simulink model "b_half_bridge_average_value_with_diode"  (R2025b)
settings: Solver=VariableStepAuto  StartTime=0.0  StopTime=1/60  RelTol=1e-3
libraries: fl_lib x19, nesl_utility x8, ee_lib x2
settings Model: SimulationMode=accelerator  Creator=gdudgeon  LastModifiedBy=gdudgeon

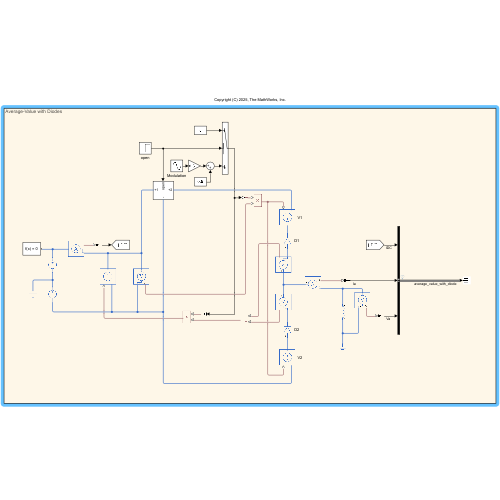
[thumbnail: Simulink's stored preview of the top-level diagram]
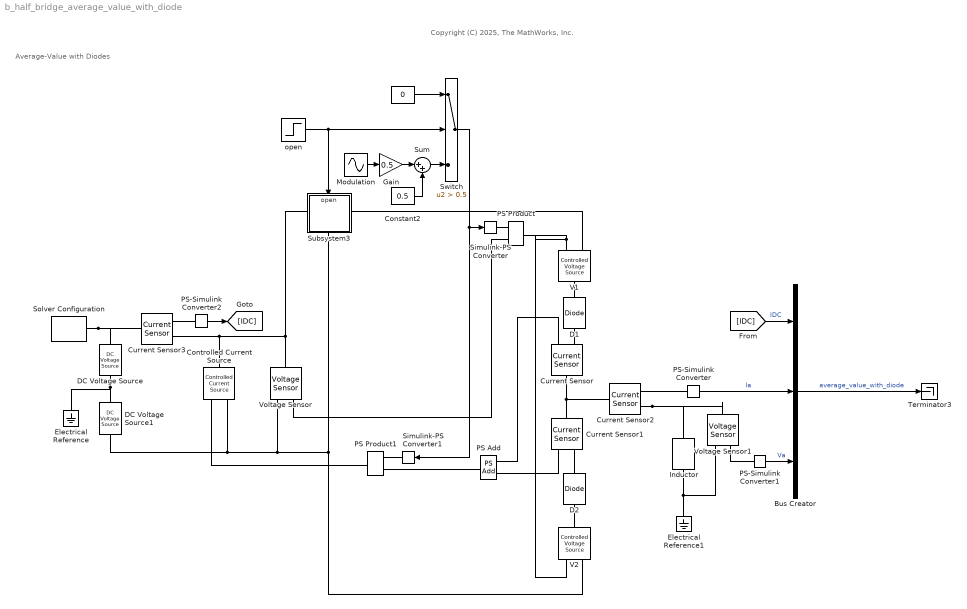
== system b_half_bridge_average_value_with_diode ==
  note: Copyright (C) 2025, The MathWorks, Inc.
  note: Average-Value with Diodes
  " " : Constant  Value=0  SampleTime=-1
  Bus Creator : BusCreator  Inputs=3
  Constant2 : Constant  Value=0.5  SampleTime=-1
  Controlled Current Source : fl_lib/Electrical/Electrical Sources/Controlled Current Source
  Current Sensor{,1..3} (4 alike) : fl_lib/Electrical/Electrical Sensors/Current Sensor
  D1 : fl_lib/Electrical/Electrical Elements/Diode  Vf=1e-3 V  Ron=1e-3 Ohm  Goff=1e-5 1/Ohm  i_specify=off  i_priority=None  i=0 A  i_nominal_specify=off  i_nominal_value=1  i_nominal_unit=A  v_specify=off  v_priority=None  v=0 V  v_nominal_specify=off  v_nominal_value=1  v_nominal_unit=V
  D2 : fl_lib/Electrical/Electrical Elements/Diode  Vf=1e-3 V  Ron=1e-3 Ohm  Goff=1e-5 1/Ohm  i_specify=off  i_priority=None  i=0 A  i_nominal_specify=off  i_nominal_value=1  i_nominal_unit=A  v_specify=off  v_priority=None  v=0 V  v_nominal_specify=off  v_nominal_value=1  v_nominal_unit=V
  DC Voltage Source : fl_lib/Electrical/Electrical Sources/DC Voltage Source  v0=50 V
  DC Voltage Source1 : fl_lib/Electrical/Electrical Sources/DC Voltage Source  v0=50 V
  Electrical Reference : fl_lib/Electrical/Electrical Elements/Electrical Reference
  Electrical Reference1 : fl_lib/Electrical/Electrical Elements/Electrical Reference
  Gain : Gain  Gain=0.5
  Inductor : fl_lib/Electrical/Electrical Elements/Inductor  l=0.01 H  r=1 Ohm  g=0 1/Ohm  i_specify=off  i_priority=None  i=0 A  i_nominal_specify=off  i_nominal_value=1  i_nominal_unit=A  v_specify=off  v_priority=High  v=0 V  v_nominal_specify=off  v_nominal_value=1  v_nominal_unit=V  i_L_specify=off  i_L_priority=High  i_L=0 A  i_L_nominal_specify=off  i_L_nominal_value=1  i_L_nominal_unit=A
  Modulation : Sin  Amplitude=0.8  Frequency=120*pi  SampleTime=0
  PS Add : fl_lib/Physical Signals/Functions/PS Add
  PS Product : fl_lib/Physical Signals/Functions/PS Product
  PS Product1 : fl_lib/Physical Signals/Functions/PS Product
  PS-Simulink Converter : nesl_utility/PS-Simulink Converter  PhysicalDomain=network_engine_domain  SubClassName=ps_output  LeftPortType=input  RightPortType=output  PseudoPeriodic=off  Frequencies=[]  VectorFormat=inherit  Unit=inherit  AffineConversion=off
  PS-Simulink Converter1 : nesl_utility/PS-Simulink Converter  PhysicalDomain=network_engine_domain  SubClassName=ps_output  LeftPortType=input  RightPortType=output  PseudoPeriodic=off  Frequencies=[]  VectorFormat=inherit  Unit=inherit  AffineConversion=off
  PS-Simulink Converter2 : nesl_utility/PS-Simulink Converter  PhysicalDomain=network_engine_domain  SubClassName=ps_output  LeftPortType=input  RightPortType=output  PseudoPeriodic=off  Frequencies=[]  VectorFormat=inherit  Unit=inherit  AffineConversion=off
  Simulink-PS Converter : nesl_utility/Simulink-PS Converter  PhysicalDomain=network_engine_domain  SubClassName=ps_input  LeftPortType=input  RightPortType=output  PseudoPeriodic=off  Frequencies=[]  NoiseDistribution=none  NoiseParameters=[]  Unit=1  AffineConversion=off  FilteringAndDerivatives=provide  SimscapeFilterOrder=1  InputFilterTimeConstant=0.001  UdotUserProvided=0
  Simulink-PS Converter1 : nesl_utility/Simulink-PS Converter  PhysicalDomain=network_engine_domain  SubClassName=ps_input  LeftPortType=input  RightPortType=output  PseudoPeriodic=off  Frequencies=[]  NoiseDistribution=none  NoiseParameters=[]  Unit=1  AffineConversion=off  FilteringAndDerivatives=provide  SimscapeFilterOrder=1  InputFilterTimeConstant=0.001  UdotUserProvided=0
  Solver Configuration : nesl_utility/Solver Configuration  PhysicalDomain=network_engine_domain  SubClassName=solver  LeftPortType=input  RightPortType=generic  Tones=[]  Harmonics=[]  SimulateNoise=off  Profile=off  UseLocalSampling=off  EnableSwitchedLinearOptims=on  FrequencyDomain=off  UseCCode=off  RelTol=0.001  AbsTol=0.001  MinStep=1e-09  ToWorkspace=off  RevertToSquareIcSolve=off  NumHomotopyIterations=100  PhasorMode=off  PhasorModeNumHarmonics=1  ConsistencySolver=NEWTON_XTOL_AFTER_FTOL  IndexReductionMethod=DerivativeReplacement  DoDC=off  ResidualTolerance=1e-09  ConsistencyTolSource=GLOBAL  ConsistencyAbsTol=0.001  ConsistencyRelTol=0.001  ConsistencyTolFactor=0.001  UseLocalSolver=on  LocalSolverChoice=NE_PARTITIONING_ADVANCER  ResolveIndetEquations=on  FunctionEvalNumThread=1  LocalSolverSampleTime=1e-6  DoFixedCost=off  MaxNonlinIter=3  MaxModeIter=2  ComputeImpulses=off  ImpulseIterations=2  LinearAlgebra=auto  LinearAlgebraNumThread=0  EquationFormulation=NE_TIME_EF  DelaysMemoryBudget=1024  AutomaticFiltering=off  FilteringTimeConstant=0.001  PartitionStorageMethod=AS_NEEDED  PartitionMemoryBudget=1024  PartitionMethod=ROBUST  MultibodyUseLocalSolver=off  MultibodyLocalSolverChoice=ODE1  MultibodyLocalSolverSampleTime=0.001
  Subsystem3 : Subsystem
      settings: PortSchema="{\"entries\":[{\"content\":{\"sides\":[{\"content\":{\"connectorIds\":[\"LConn1\"]},\"type\":\"ConnectorPlacement.EquallySpacedRectSide\",\"uuid\":\"88db1bd8-f64b-4165-8d2c-7cfa4014cba2\"},{\"content\":{\"connectorIds\":[\"RConn1\"],\"side\":\"RIGHT\"},\"type\":\"ConnectorPlacement.EquallySpacedRectSide\",\"uuid\":\"19f0c499-9eed-48d3-a8f5-fe9dad581b85\"},{\"content\":{\"connectorIds\":[\"In1\"],\"side\":\"TOP\"},\"type\":\"ConnectorPlacement.EquallySpacedRectSide\",\"uuid\":\"71d5fe89-ffc2-4430-819d-512bfd197a1c\"},{\"content\":{\"connectorIds\":[\"RConn2\"],\"side\":\"BOTTOM\"},\"type\":\"ConnectorPlacement.EquallySpacedRectSide\",\"uuid\":\"b828cb58-5f78-4b23-b8a0-147c7a9d81e7\"}]},\"type\":\"ConnectorPlacement.EquallySpacedConnector\",\"uuid\":\"64b174d4-80a0-4eb7-9a75-e3677787263f\"}],\"packageUris\":[\"http://schema.mathworks.com/mf0/Connector/R2020b\"],\"version\":\"1.0\"}"
  Sum : Sum  Inputs=|++
  Switch : Switch  Criteria=u2 > Threshold  Threshold=0.5  SaturateOnIntegerOverflow=off  InputSameDT=off
  Terminator3 : Terminator
  V1 : fl_lib/Electrical/Electrical Sources/Controlled Voltage Source
  V2 : fl_lib/Electrical/Electrical Sources/Controlled Voltage Source
  Voltage Sensor : fl_lib/Electrical/Electrical Sensors/Voltage Sensor
  Voltage Sensor1 : fl_lib/Electrical/Electrical Sensors/Voltage Sensor
  open : Step  After=0  SampleTime=0
  wires:
  Switch/1 -> Simulink-PS Converter1/1, Simulink-PS Converter/1
  " "/1 -> Switch/1
  [IDC] -> Bus Creator/1  "IDC"
  PS-Simulink Converter2/1 -> [IDC]
  open/1 -> Switch/2, Subsystem3/1(open)
  Bus Creator/1 -> Terminator3/1  "average_value_with_diode"
  PS-Simulink Converter1/1 -> Bus Creator/3  "Va"
  PS-Simulink Converter/1 -> Bus Creator/2  "Ia"
  Sum/1 -> Switch/3
  Modulation/1 -> Gain/1
  Constant2/1 -> Sum/2
  Gain/1 -> Sum/1
  connections:
  Solver Configuration/RConn1 -- DC Voltage Source/LConn1 -- Current Sensor3/LConn1
  Current Sensor3/RConn2 -- Controlled Current Source/LConn1 -- Subsystem3/LConn1 -- Voltage Sensor/LConn1
  Current Sensor2/LConn1 -- Current Sensor1/LConn1 -- Current Sensor/LConn1
  Electrical Reference1/LConn1 -- Inductor/RConn1 -- Voltage Sensor1/RConn2
  DC Voltage Source/RConn1 -- DC Voltage Source1/LConn1 -- Electrical Reference/LConn1
  Current Sensor2/RConn2 -- Inductor/LConn1 -- Voltage Sensor1/LConn1
  V1/RConn1 -- V2/RConn1 -- PS Product/RConn1
  Subsystem3/RConn2 -- V2/RConn2 -- Voltage Sensor/RConn2 -- DC Voltage Source1/RConn1 -- Controlled Current Source/RConn2
  Voltage Sensor/RConn1 -- PS Product/LConn2
  PS Add/LConn1 -- Current Sensor1/RConn1
  D2/LConn1 -- V2/LConn1
  Simulink-PS Converter/RConn1 -- PS Product/LConn1
  PS-Simulink Converter2/LConn1 -- Current Sensor3/RConn1
  D1/RConn1 -- V1/LConn1
  PS Product1/LConn1 -- PS Add/RConn1
  D1/LConn1 -- Current Sensor/RConn2
  PS Product1/RConn1 -- Controlled Current Source/RConn1
  PS-Simulink Converter1/LConn1 -- Voltage Sensor1/RConn1
  Subsystem3/RConn1 -- V1/RConn2
  Simulink-PS Converter1/RConn1 -- PS Product1/LConn2
  D2/RConn1 -- Current Sensor1/RConn2
  Current Sensor2/RConn1 -- PS-Simulink Converter/LConn1
  PS Add/LConn2 -- Current Sensor/RConn1

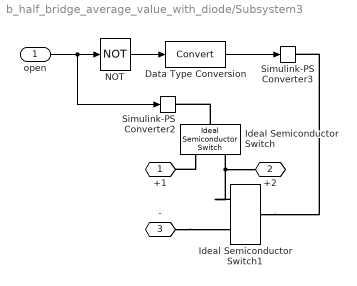
== system b_half_bridge_average_value_with_diode/Subsystem3 ==
  open : Inport
  Data Type Conversion : DataTypeConversion  SaturateOnIntegerOverflow=off  RndMeth=Floor
  Ideal Semiconductor Switch : ee_lib/Semiconductors & Converters/Ideal Semiconductor Switch  port_option=ee.enum.controlport.ps  Ron=1e-5 Ohm  Goff=1e-5 1/Ohm  Vth=0.5 V  diode_param=ee.enum.semiconductors.protectionDiode.external  diode_Vf=0.8 V  diode_Ron=0.001 Ohm  diode_Goff=1e-5 1/Ohm  diode_C=50e-9 F  diode_iRM=-235 A  diode_iF=300 A  diode_idot=-50 A/us  diode_trr_param=ee.enum.converters.diodetrr.trr_factor  diode_trr_factor=3  diode_trr=15 us  diode_Qrr=1500 s*uA
  Ideal Semiconductor Switch1 : ee_lib/Semiconductors & Converters/Ideal Semiconductor Switch  port_option=ee.enum.controlport.ps  Ron=1e-5 Ohm  Goff=1e-5 1/Ohm  Vth=0.5 V  diode_param=ee.enum.semiconductors.protectionDiode.external  diode_Vf=0.8 V  diode_Ron=0.001 Ohm  diode_Goff=1e-5 1/Ohm  diode_C=50e-9 F  diode_iRM=-235 A  diode_iF=300 A  diode_idot=-50 A/us  diode_trr_param=ee.enum.converters.diodetrr.trr_factor  diode_trr_factor=3  diode_trr=15 us  diode_Qrr=1500 s*uA
  NOT : Logic  Operator=NOT  IconShape=distinctive  AllPortsSameDT=off  OutDataTypeStr=boolean
  Simulink-PS Converter2 : nesl_utility/Simulink-PS Converter  PhysicalDomain=network_engine_domain  SubClassName=ps_input  LeftPortType=input  RightPortType=output  PseudoPeriodic=off  Frequencies=[]  NoiseDistribution=none  NoiseParameters=[]  Unit=1  AffineConversion=off  FilteringAndDerivatives=provide  SimscapeFilterOrder=1  InputFilterTimeConstant=0.001  UdotUserProvided=0
  Simulink-PS Converter3 : nesl_utility/Simulink-PS Converter  PhysicalDomain=network_engine_domain  SubClassName=ps_input  LeftPortType=input  RightPortType=output  PseudoPeriodic=off  Frequencies=[]  NoiseDistribution=none  NoiseParameters=[]  Unit=1  AffineConversion=off  FilteringAndDerivatives=provide  SimscapeFilterOrder=1  InputFilterTimeConstant=0.001  UdotUserProvided=0
  +1 : PMIOPort  Side=Left
  +2 : PMIOPort  Port=2  Side=Right
  - : PMIOPort  Port=3  Side=Right
  wires:
  Data Type Conversion/1 -> Simulink-PS Converter3/1
  NOT/1 -> Data Type Conversion/1
  open/1 -> NOT/1, Simulink-PS Converter2/1
  connections:
  Ideal Semiconductor Switch/RConn2 -- +1/RConn1
  Ideal Semiconductor Switch/LConn1 -- Simulink-PS Converter2/RConn1
  Ideal Semiconductor Switch1/RConn2 -- Ideal Semiconductor Switch/RConn1 -- +2/RConn1
  Ideal Semiconductor Switch1/LConn1 -- Simulink-PS Converter3/RConn1
  -/RConn1 -- Ideal Semiconductor Switch1/RConn1
